simulink model "Simulink_Model"  (R2026a)
settings: Solver=VariableStepAuto  StopTime=5
InitFcn:
  | Iy = 2.43e6;
  | m = 5830;
  | T = 341000;
  | F = 375000;
  | x_cp = 38;
  | x_cg = 32.3;
  | V = 1320;
  | V_w = 132;
  | alpha_w = 5.73*pi/180;
  | N_alpha = 240000;
  | M_alpha = 3.75;
  | M_delta = 4.54;
settings Model: Creator=Dheeraj  LastModifiedBy=Dheeraj

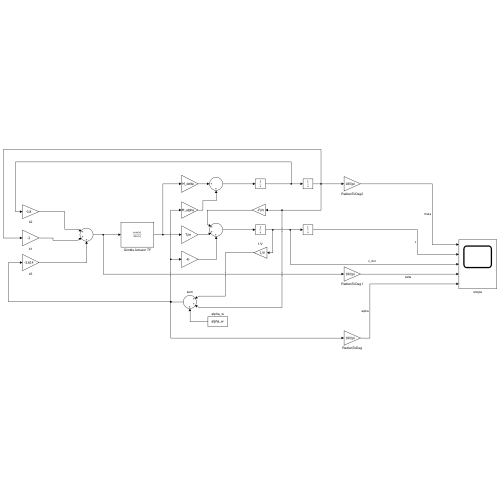
[thumbnail: Simulink's stored preview of the top-level diagram]
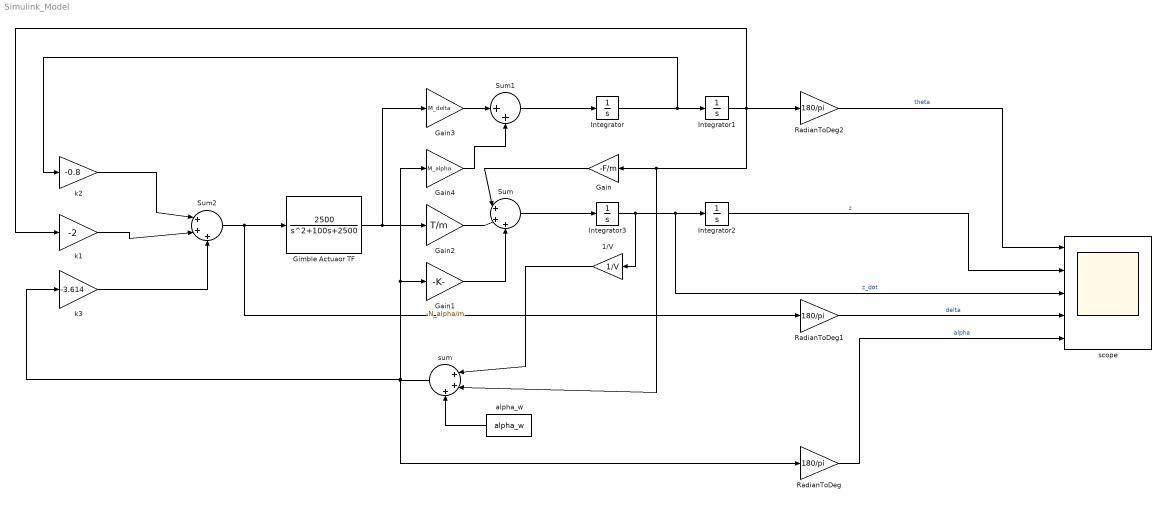
== system Simulink_Model ==
  1/V : Gain  Gain=1/V
  Gain : Gain  Gain=-F/m
  Gain1 : Gain  Gain=-N_alpha/m
  Gain2 : Gain  Gain=T/m
  Gain3 : Gain  Gain=M_delta
  Gain4 : Gain  Gain=M_alpha
  Gimble Actuaor TF : TransferFcn  Numerator=[2500]  Denominator=[1 100 2500]
  Integrator{,1..3} (4 alike) : Integrator
  RadianToDeg : Gain  Gain=180/pi
  RadianToDeg1 : Gain  Gain=180/pi
  RadianToDeg2 : Gain  Gain=180/pi
  Sum : Sum  Inputs=|+++
  Sum1 : Sum  Inputs=|++
  Sum2 : Sum  Inputs=|+++
  alpha_w : Constant  Value=alpha_w
  k1 : Gain  Gain=-2
  k2 : Gain  Gain=-0.8
  k3 : Gain  Gain=-3.614
  scope : Scope  NumInputPorts=5
      settings: ActiveDisplayYMinimum=-24.375582598729448  ActiveDisplayYMaximum=10.464760936013853
  sum : Sum  Inputs=|+++
  wires:
  Integrator/1 -> Integrator1/1, k2/1
  Integrator1/1 -> Gain/1, sum/2, RadianToDeg2/1, k1/1
  Gain/1 -> Sum/1
  Sum/1 -> Integrator3/1
  alpha_w/1 -> sum/3
  1/V/1 -> sum/1
  sum/1 -> Gain4/1, Gain1/1, k3/1, RadianToDeg/1
  Gain1/1 -> Sum/3
  Gain2/1 -> Sum/2
  Sum1/1 -> Integrator/1
  Gain3/1 -> Sum1/1
  Gain4/1 -> Sum1/2
  Gimble Actuaor TF/1 -> Gain3/1, Gain2/1
  Integrator2/1 -> scope/2  "z"
  Sum2/1 -> RadianToDeg1/1, Gimble Actuaor TF/1
  k1/1 -> Sum2/2
  k2/1 -> Sum2/1
  k3/1 -> Sum2/3
  Integrator3/1 -> 1/V/1, scope/3, Integrator2/1  "z_dot"
  RadianToDeg2/1 -> scope/1  "theta"
  RadianToDeg1/1 -> scope/4  "delta"
  RadianToDeg/1 -> scope/5  "alpha"
